simulink model "nms_3Dmodel_forward_no_rbld"  (R2017b)
settings: Solver=VariableStepAuto  StartTime=0.0  StopTime=t_end  FixedStep=1e-4  MinStep=1e-9  RelTol=1e-2  AbsTol=1e-3  EnableMultiTasking=on
InitFcn:
  | runScripts;
values from neighbouring files (symbols this model uses):
  ankle_height = 0.08    [nms_MechInit.m]
  ankleIMP = param(91+length(paramIC_opt):93+length(paramIC_opt))    [runScripts.m]
  c = 0.05    [IID_nms_MechInit.m]    (also in nms_MechInit.m)
  c_jointstop = 0.3 / (pi/180)    (= 17.1887338539)    [IID_nms_MechInit.m]    (also in nms_MechInit.m)
  CPG_On = 0    [setCPGPar.m]    (also in setCPGPar_inv.m = 1)
  CtrlPar_FP = [alpha0 alpha_cd alpha_cv]    [setCtrlPar.m]
  CtrlPar_FP_R = [R_hipR0 R_hipR_cd R_hipR_cv]    [setCtrlPar.m]
  CtrlPar_LL = l_clr    [setCtrlPar.m]
  CtrlPar_Side = [beta_cd  beta_cv]    [setCtrlPar.m]
  CtrlPar_St = [StPreStim St_M1 St_M2 St_M3 St_M4 St_M5 St_M11]    [setCtrlPar.m]
  CtrlPar_St_R = [R_StPreStim R_St_M1 R_St_M3 R_St_M4]    [setCtrlPar.m]
  CtrlPar_Sw = [SwPreStim SwPhasePari SwPhaseParii SwCtrlPar_H SwCtrlPar_A      SwCtrlPar_Ki SwCtrlPar_Kii SwCtrlPar_Kiii SwCtrlPar_StP]    [setCtrlPar.m]
  CtrlPar_Sw_R = [R_SwPreStim R_Sw_M6]    [setCtrlPar.m]
  CtrlPar_theta0 = parBlCtrl(1)      *1*pi/180    [setCtrlPar.m]
  CtrlPar_Tr = [Tr_St_sup Tr_Sw]    [setCtrlPar.m]
  CtrlPar_Tr_R = [R_Tr_St_sup R_Tr_Sw]    [setCtrlPar.m]
  D12_F = 0.16    [IID_nms_MechInit.m]    (also in nms_MechInit.m)
  D12_S = L_S    (= 0.5)    [IID_nms_MechInit.m]    (also in nms_MechInit.m = 0.46)
  D12_T = L_T    (= 0.5)    [IID_nms_MechInit.m]    (also in nms_MechInit.m = 0.46)
  D12z_T = 0.1* scalorFactor    (= 0.1)    [nms_MechInit.m]
  D13_F = 0.20    (= 0.2)    [IID_nms_MechInit.m]    (also in nms_MechInit.m)
  D1G_F = 0.14    [IID_nms_MechInit.m]    (also in nms_MechInit.m)
  D1G_HAT = 0.35    [IID_nms_MechInit.m]    (also in nms_MechInit.m)
  D1G_S = 0.3    [IID_nms_MechInit.m]    (also in nms_MechInit.m = 0.28)
  D1G_T = 0.3    [IID_nms_MechInit.m]    (also in nms_MechInit.m = 0.28)
  D1Gy_F = ankle_height*D1G_F/D12_F    (= 0.07)    [nms_MechInit.m]
  d_fBall = 0.1    [nms_MechInit.m]
  d_fHeel = 0.05    [nms_MechInit.m]
  DeltaThRef = 5e-3    (= 0.005)    [IID_nms_MechInit.m]    (also in nms_MechInit.m)
  Dist_LM23_PH = 0    [setDistPar.m]
  Dist_LM34_PH = 0    [setDistPar.m]
  Dist_On = 1    [IID_setDistPar.m]    (also in setDistPar.m)
  Dist_PDur = 0.15    [IID_setDistPar.m]    (also in setDistPar.m)
  Dist_RM23_PH = 0    [setDistPar.m]
  Dist_RM34_PH = 0    [setDistPar.m]
  Dist_StartTime = 15    [IID_setDistPar.m]    (also in setDistPar.m)
  Dist_xyzHAT_front_PH = 0    [setDistPar.m]
  Dist_xyzHAT_sag_PH = 0    [IID_setDistPar.m]    (also in setDistPar.m)
  Dist_xyzLAnkle_PH = 0    [setDistPar.m]
  Dist_xyzRAnkle_PH = 0    [setDistPar.m]
  eref = 0.04    [IID_nms_MechInit.m]    (also in nms_MechInit.m)
  FmaxBFSH = 350    [nms_MechInit.m]
  FmaxGAS = 1500    [IID_nms_MechInit.m]    (also in nms_MechInit.m)
  FmaxGLU = 1500    [IID_nms_MechInit.m]    (also in nms_MechInit.m)
  FmaxHAB = 3000    [nms_MechInit.m]
  FmaxHAD = 4500    [nms_MechInit.m]
  FmaxHAM = 3000    [IID_nms_MechInit.m]    (also in nms_MechInit.m)
  FmaxHFL = 2000    [IID_nms_MechInit.m]    (also in nms_MechInit.m)
  FmaxRF = 1200    [nms_MechInit.m]
  FmaxSOL = 4000    [IID_nms_MechInit.m]    (also in nms_MechInit.m)
  FmaxTA = 800    [IID_nms_MechInit.m]    (also in nms_MechInit.m)
  FmaxVAS = 6000    [IID_nms_MechInit.m]    (also in nms_MechInit.m)
  In_F = 0.005    [IID_nms_MechInit.m]    (also in nms_MechInit.m)
  In_HAT = 3    [IID_nms_MechInit.m]    (also in nms_MechInit.m = 2.5)
  In_S = 0.05    [IID_nms_MechInit.m]    (also in nms_MechInit.m)
  In_T = 0.15    [IID_nms_MechInit.m]    (also in nms_MechInit.m)
  init_a_tgt = 70*pi/180    (= 1.2217304764)    [setInitPar.m]
  init_a_tgtR = 90*pi/180    (= 1.57079632679)    [setInitPar.m]
  Inx_F = 0.0007    [nms_MechInit.m]
  Inx_HAT = 1.0    (= 1)    [nms_MechInit.m]
  Inx_S = 0.003    [nms_MechInit.m]
  Inx_T = 0.03    [nms_MechInit.m]
  Iny_F = 0.005    [nms_MechInit.m]
  Iny_HAT = 4.0    (= 4)    [nms_MechInit.m]
  Iny_S = 0.05    [nms_MechInit.m]
  Iny_T = 0.15    [nms_MechInit.m]
  K = 5    [IID_nms_MechInit.m]    (also in nms_MechInit.m)
  k_gn = k_gn/2    (= 39240)    [nms_MechInit.m]
  k_gt = k_gt/2    (= 3924)    [nms_MechInit.m]
  k_pressure = m_HAT * 9.81 / DeltaThRef    (= 104967)    [IID_nms_MechInit.m]    (also in nms_MechInit.m)
  leg_l = [D12_T D12_S]    [nms_MechInit.m]
  LongDelay = 0.020    (= 0.02)    [IID_setCtrlPar.m]    (also in nms_MechInit.m = 0.01)
  LongLoopDelay = 0.030    (= 0.03)    [nms_MechInit.m]
  loptBFSH = 0.12    [nms_MechInit.m]
  loptGAS = 0.05    [IID_nms_MechInit.m]    (also in nms_MechInit.m)
  loptGLU = 0.11    [IID_nms_MechInit.m]    (also in nms_MechInit.m)
  loptHAB = 0.09    [nms_MechInit.m]
  loptHAD = 0.10    (= 0.1)    [nms_MechInit.m]
  loptHAM = 0.10    (= 0.1)    [IID_nms_MechInit.m]    (also in nms_MechInit.m)
  loptHFL = 0.11    [IID_nms_MechInit.m]    (also in nms_MechInit.m)
  loptRF = 0.08    [nms_MechInit.m]
  loptSOL = 0.04    [IID_nms_MechInit.m]    (also in nms_MechInit.m)
  loptTA = 0.06    [IID_nms_MechInit.m]    (also in nms_MechInit.m)
  loptVAS = 0.08    [IID_nms_MechInit.m]    (also in nms_MechInit.m)
  lslackBFSH = 0.10    (= 0.1)    [nms_MechInit.m]
  lslackGAS = 0.40    (= 0.4)    [IID_nms_MechInit.m]    (also in nms_MechInit.m)
  lslackGLU = 0.13    [IID_nms_MechInit.m]    (also in nms_MechInit.m)
  lslackHAB = 0.07    [nms_MechInit.m]
  lslackHAD = 0.18    [nms_MechInit.m]
  lslackHAM = 0.31    [IID_nms_MechInit.m]    (also in nms_MechInit.m)
  lslackHFL = 0.10    (= 0.1)    [IID_nms_MechInit.m]    (also in nms_MechInit.m)
  lslackRF = 0.35    [nms_MechInit.m]
  lslackSOL = 0.26    [IID_nms_MechInit.m]    (also in nms_MechInit.m)
  lslackTA = 0.24    [IID_nms_MechInit.m]    (also in nms_MechInit.m)
  lslackVAS = 0.23    [IID_nms_MechInit.m]    (also in nms_MechInit.m)
  m_F = 1.25    [IID_nms_MechInit.m]    (also in nms_MechInit.m)
  m_HAT = 53.5    [IID_nms_MechInit.m]    (also in nms_MechInit.m)
  m_S = 3.5    [IID_nms_MechInit.m]    (also in nms_MechInit.m)
  m_T = 8.5    [IID_nms_MechInit.m]    (also in nms_MechInit.m)
  m_Total = m_F*2+m_S*2+m_T*2+m_HAT    (= 80)    [IID_nms_MechInit.m]    (also in nms_MechInit.m)
  massBFSH = 2    [nms_MechInit.m]
  massGAS = 0.45    [IID_nms_MechInit.m]    (also in nms_MechInit.m)
  massGLU = 1.4    [IID_nms_MechInit.m]    (also in nms_MechInit.m)
  massHAB = 1.145    [nms_MechInit.m]
  massHAD = 1.91    [nms_MechInit.m]
  massHAM = 1.82    [IID_nms_MechInit.m]    (also in nms_MechInit.m)
  massHFL = 1.87    [IID_nms_MechInit.m]    (also in nms_MechInit.m)
  massRF = 1    [nms_MechInit.m]
  massSOL = 1.36    [IID_nms_MechInit.m]    (also in nms_MechInit.m)
  massTA = 0.29    [IID_nms_MechInit.m]    (also in nms_MechInit.m)
  massVAS = 2.91    [IID_nms_MechInit.m]    (also in nms_MechInit.m)
  MidDelay = 0.010    (= 0.01)    [IID_setCtrlPar.m]    (also in nms_MechInit.m = 0.005)
  mu_slide = 0.8    [IID_nms_MechInit.m]    (also in nms_MechInit.m)
  mu_stick = 0.9    [IID_nms_MechInit.m]    (also in nms_MechInit.m)
  N = 1.5    [IID_nms_MechInit.m]    (also in cmaes_parfor.m = size(x,1); nms_MechInit.m)
  phi12_LowLimit = 70*pi/180    (= 1.2217304764)    [IID_nms_MechInit.m]    (also in nms_MechInit.m)
  phi12_UpLimit = 130*pi/180    (= 2.26892802759)    [IID_nms_MechInit.m]    (also in nms_MechInit.m)
  phi23_UpLimit = 175*pi/180    (= 3.05432619099)    [IID_nms_MechInit.m]    (also in nms_MechInit.m)
  phi34_UpLimit = 230*pi/180    (= 4.01425727959)    [IID_nms_MechInit.m]    (also in nms_MechInit.m)
  phi34R_LowLimit = -15*pi/180    (= -0.261799387799)    [nms_MechInit.m]
  ... (+115 more)
undefined symbols (not defined in the file or in its folder): magnitude, sgn
libraries: mblibv1 x104, simulink x54, simulink_extras x38, nmc x30, NMCCPG_Library x17, powerlib_meascontrol x5
(part 15 of 17)

== system nms_3Dmodel_forward_no_rbld/Neural Control Layer (Spinal Cord Control)/R Swing Phase (sagittal)/kneeii_damp and hold &kneeiii_leg stop &kneeiv_stance preparation ==
  note: Knee Phase i
  CtrlPar : Inport
  a_tgt : Inport  Port=2
  LceRF : Inport  Port=3
  LceHAM : Inport  Port=4
  VceHAM : Inport  Port=5
  VceVAS : Inport  Port=6
  VceBFSH : Inport  Port=7
  VceRF : Inport  Port=8
  LceHFL : Inport  Port=9
  LceGLU : Inport  Port=10
  LceVAS : Inport  Port=11
  Enable : EnablePort  StatesWhenEnabling=reset  ZeroCross=off
  Compare To Constant : simulink/Logic and Bit Operations/Compare To Constant  relop=<=  const=0  OutDataTypeStr=uint8  ZeroCross=off
  Constant1 : Constant  Value=0  OutDataTypeStr=boolean
  Constant2 : Constant  Value=0  OutDataTypeStr=boolean
  Constant3 : Constant  Value=0  OutDataTypeStr=boolean
  Constant4 : Constant
  Constant5 : Constant
  Demux1 : Demux  Outputs=5
  Divide1 : Product
  Divide2 : Product
  Logical Operator : Logic  Operator=NOT  AllPortsSameDT=off  OutDataTypeStr=boolean
  Logical Operator1 : Logic  AllPortsSameDT=off  OutDataTypeStr=boolean
  Relational Operator : RelationalOperator  Operator=<=  OutDataTypeStr=boolean  ZeroCross=off  RndMeth=Nearest
  Relational Operator1 : RelationalOperator  OutDataTypeStr=boolean  ZeroCross=off  RndMeth=Nearest
  S-R Flip-Flop : simulink_extras/Flip Flops/S-R Flip-Flop  initial_condition=0
  S-R Flip-Flop1 : simulink_extras/Flip Flops/S-R Flip-Flop  initial_condition=0
  S-R Flip-Flop2 : simulink_extras/Flip Flops/S-R Flip-Flop  initial_condition=0
  Sum1 : Sum  Inputs=+-|  SaturateOnIntegerOverflow=on  InputSameDT=on  OutDataTypeStr=Inherit: Same as first input
  Sum2 : Sum  Inputs=++|  SaturateOnIntegerOverflow=on  InputSameDT=on  OutDataTypeStr=Inherit: Same as first input
  Sum3 : Sum  Inputs=+-|  SaturateOnIntegerOverflow=on  InputSameDT=on  OutDataTypeStr=Inherit: Same as first input
  Sum4 : Sum  Inputs=+-|  SaturateOnIntegerOverflow=on  InputSameDT=on  OutDataTypeStr=Inherit: Same as first input
  Sum5 : Sum  Inputs=++|  SaturateOnIntegerOverflow=on  InputSameDT=on  OutDataTypeStr=Inherit: Same as first input
  Terminator : Terminator
  Terminator1 : Terminator
  Terminator2 : Terminator
  kneeii_damp and hold : Subsystem  TreatAsAtomicUnit=on
  kneeiii_leg stop : Subsystem  TreatAsAtomicUnit=on
  kneeiv_stance preparation : Subsystem  TreatAsAtomicUnit=on
  parSwKii : Selector  InputPortWidth=Sw_i  IndexOptions=Index vector (dialog)  Indices=parSwKii_i  OutputSizes=1
  parSwKiii : Selector  InputPortWidth=Sw_i  IndexOptions=Index vector (dialog)  Indices=parSwKiii_i  OutputSizes=1
  parSwKiv : Selector  InputPortWidth=Sw_i  IndexOptions=Index vector (dialog)  Indices=parSwKiv_i  OutputSizes=1
  parSwPhii : Selector  InputPortWidth=Sw_i  IndexOptions=Index vector (dialog)  Indices=parSwPhii_i  OutputSizes=1
  SRF_Sw_kii : Outport  OutputWhenDisabled=reset  InitialOutput=0
  SBFSH_Sw_kii : Outport  Port=2  OutputWhenDisabled=reset  InitialOutput=0
  SHAM_Sw_kiii : Outport  Port=3  OutputWhenDisabled=reset  InitialOutput=0
  SBFSH_Sw_kiii : Outport  Port=4  OutputWhenDisabled=reset  InitialOutput=0
  SGAS_Sw_kiii : Outport  Port=5  OutputWhenDisabled=reset  InitialOutput=0
  SHFL_Sw_kiv : Outport  Port=6  OutputWhenDisabled=reset  InitialOutput=0
  SGLU_Sw_kiv : Outport  Port=7  OutputWhenDisabled=reset  InitialOutput=0
  SVAS_Sw_kiv : Outport  Port=8  OutputWhenDisabled=reset  InitialOutput=0
  wires:
  Constant1/1 -> S-R Flip-Flop/2
  S-R Flip-Flop/2 -> Terminator/1
  Relational Operator/1 -> S-R Flip-Flop/1
  Constant2/1 -> S-R Flip-Flop1/2
  S-R Flip-Flop1/2 -> Terminator1/1
  Relational Operator1/1 -> S-R Flip-Flop1/1
  Constant3/1 -> S-R Flip-Flop2/2
  S-R Flip-Flop2/2 -> Terminator2/1
  Logical Operator1/1 -> S-R Flip-Flop2/1
  CtrlPar/1 -> parSwKii/1, parSwKiii/1, parSwKiv/1, parSwPhii/1
  S-R Flip-Flop/1 -> Logical Operator/1
  parSwKii/1 -> kneeii_damp and hold/1(CtrlPar)
  S-R Flip-Flop1/1 -> kneeiii_leg stop/Enable, Logical Operator1/1
  S-R Flip-Flop2/1 -> kneeiv_stance preparation/Enable
  parSwKiii/1 -> kneeiii_leg stop/1(CtrlPar)
  parSwKiv/1 -> kneeiv_stance preparation/1(CtrlPar)
  kneeii_damp and hold/1(SRF_Sw_kii) -> SRF_Sw_kii/1
  kneeii_damp and hold/2(SBFSH_Sw_kii) -> SBFSH_Sw_kii/1
  kneeiii_leg stop/1(SHAM_Sw_kiii) -> SHAM_Sw_kiii/1
  kneeiii_leg stop/2(SKFL_Sw_kiii) -> SBFSH_Sw_kiii/1
  kneeiii_leg stop/3(SGAS_Sw_kiii) -> SGAS_Sw_kiii/1
  kneeiv_stance preparation/1(SHFL_Sw_kiv) -> SHFL_Sw_kiv/1
  kneeiv_stance preparation/2(SGLU_Sw_kiv) -> SGLU_Sw_kiv/1
  kneeiv_stance preparation/3(SVAS_Sw_kiv) -> SVAS_Sw_kiv/1
  parSwPhii/1 -> Demux1/1
  Demux1/1 -> Sum3/2  "aRef_RF"
  Sum3/1 -> Divide1/1
  Constant4/1 -> Sum5/1
  Divide1/1 -> Sum5/2
  a_tgt/1 -> Sum2/1, Sum3/1, kneeii_damp and hold/2(a_tgt), kneeiii_leg stop/2(a_tgt), kneeiv_stance preparation/2(a_tgt)
  Demux1/2 -> Divide1/2  "a2lopt_RF"
  Sum5/1 -> Relational Operator/2  "lceOffRF"
  LceRF/1 -> kneeii_damp and hold/6(LceRF), Relational Operator/1
  Logical Operator/1 -> kneeii_damp and hold/Enable
  Demux1/3 -> Sum2/2  "a_del"
  Sum2/1 -> Sum1/1  "a_thr"
  Demux1/4 -> Sum1/2  "aRef_HAM"
  Sum1/1 -> Divide2/1
  Demux1/5 -> Divide2/2  "a2lopt_HAM"
  Constant5/1 -> Sum4/1
  Divide2/1 -> Sum4/2
  Sum4/1 -> Relational Operator1/2  "lceOffHAM"
  LceHAM/1 -> kneeiii_leg stop/3(LceHAM), Relational Operator1/1  "LceHAM"
  Compare To Constant/1 -> Logical Operator1/2
  VceHAM/1 -> Compare To Constant/1
  VceBFSH/1 -> kneeii_damp and hold/4(VceBFSH)
  VceRF/1 -> kneeii_damp and hold/5(VceRF)
  LceHFL/1 -> kneeiv_stance preparation/3(LceHFL)
  LceGLU/1 -> kneeiv_stance preparation/4(lceGLU)
  LceVAS/1 -> kneeiv_stance preparation/5(lceVAS)
  VceVAS/1 -> kneeii_damp and hold/3(VceVAS)

== system nms_3Dmodel_forward_no_rbld/Body Mechanics Layer/LLHeelCnt1/3D Contact/Friction Switch ==
  note: Static/Kinetic Friction Switch
  Slide! : Inport
  Stick! : Inport  Port=2
  Memory : Memory
  S-R Flip-Flop : simulink_extras/Flip Flops/S-R Flip-Flop  initial_condition=0
  Terminator : Terminator
  Stiction : Outport
  wires:
  Memory/1 -> Stiction/1
  Slide!/1 -> S-R Flip-Flop/2
  Stick!/1 -> S-R Flip-Flop/1
  S-R Flip-Flop/2 -> Terminator/1
  S-R Flip-Flop/1 -> Memory/1

== system nms_3Dmodel_forward_no_rbld/Body Mechanics Layer/LLHeelCnt1/3D Contact/Kinetic Friction Model ==
  note: Tangential Ground Friction
  note: Normal Ground Friction
  note: Sliding Limit Detector
  note: Footpoint Determiner
  note: Kinetic Friction Model
  vel [m/s m/s m/s] : Inport
  pos [m m m] : Inport  Port=2
  RefPt [m m m] : Inport  Port=3
  nVec [m m m] : Inport  Port=4
  Enable : EnablePort  StatesWhenEnabling=reset  ZeroCross=off
  Constant : Constant  Value=vLimit
  Constant1 : Constant  Value=[0 0 0 1]'
  Demux : Demux  Outputs=[3 1]
  FixPt Relational Operator : RelationalOperator  Operator=>  OutDataTypeStr=boolean  ZeroCross=off  RndMeth=Nearest
  Gain3 : Gain  Gain=k_gn
  Gain4 : Gain  Gain=1/v_gn_max
  Memory : Memory
  Mux1 : Mux  Inputs=2
  Mux2 : Mux  Inputs=2
  Negative : simulink/Logic and Bit Operations/Compare To Zero  relop=<  OutDataTypeStr=boolean
  Normal Axis Ground Force : Fcn  Expr="u(1)  *  (1-u(2)) * (u(2)<1)"
  Product : Product  RndMeth=Zero
  Product1 : Product  RndMeth=Zero
  Sum : Sum  Inputs=|+-
  Switch : Switch  Criteria=u2 > Threshold  Threshold=0.9*vLimit
      settings: AttributesFormatString=>%<Threshold>?
  Vector Norm : Subsystem
  d_n : DotProduct  InputSameDT=on  OutDataTypeStr=Inherit: Inherit via internal rule
  qnVec : Sum  Inputs=-+
  reverse direction : Gain  Gain=-1
  sliding friction coefficient : Gain  Gain=mu_slide
  tVec : Product  Inputs=*/  RndMeth=Zero
  v_n : DotProduct  InputSameDT=on  OutDataTypeStr=Inherit: Inherit via internal rule
  v_nVec : Product  RndMeth=Zero
  v_tVec : Sum  Inputs=-+|
  RefPtFP [m m m] : Outport  InitialOutput=[0 0 0]
      settings: AttributesFormatString=initial = '%<InitialOutput>'\nwhen disabled = '%<OutputWhenDisabled>'
  posFP [m m m] : Outport  Port=2  InitialOutput=[0 0 0]
      settings: AttributesFormatString=initial = '%<InitialOutput>'\nwhen disabled = '%<OutputWhenDisabled>'
  nVec FP [m m m] : Outport  Port=3  InitialOutput=0
      settings: AttributesFormatString=initial = '%<InitialOutput>'\nwhen disabled = '%<OutputWhenDisabled>'
  Stiction! : Outport  Port=4  OutputWhenDisabled=reset  InitialOutput=0
      settings: AttributesFormatString=initial = '%<InitialOutput>'\nwhen disabled = '%<OutputWhenDisabled>'
  F_t Slide [N N N] : Outport  Port=5  OutputWhenDisabled=reset  InitialOutput=[0 0 0]
      settings: AttributesFormatString=initial = '%<InitialOutput>'\nwhen disabled = '%<OutputWhenDisabled>'
  F_n Slide [N N N] : Outport  Port=6  OutputWhenDisabled=reset  InitialOutput=[0 0 0]
      settings: AttributesFormatString=initial = '%<InitialOutput>'\nwhen disabled = '%<OutputWhenDisabled>'
  wires:
  RefPt [m m m]/1 -> RefPtFP [m m m]/1, qnVec/2
  qnVec/1 -> d_n/1
  pos [m m m]/1 -> qnVec/1, posFP [m m m]/1
  Demux/1 -> tVec/1
  Demux/2 -> tVec/2
  Switch/1 -> Demux/1
  Mux2/1 -> Switch/1
  Constant1/1 -> Switch/3
  tVec/1 -> reverse direction/1
  Product1/1 -> F_n Slide [N N N]/1
  reverse direction/1 -> Product/2
  sliding friction coefficient/1 -> Product/1
  v_tVec/1 -> Mux2/1, Vector Norm/1(vec)
  v_nVec/1 -> v_tVec/1
  v_n/1 -> v_nVec/1, Gain4/1
  vel [m/s m/s m/s]/1 -> v_tVec/2, v_n/2
  d_n/1 -> Gain3/1
  nVec [m m m]/1 -> nVec FP [m m m]/1, Product1/1, d_n/2, v_nVec/2, v_n/1
  Gain4/1 -> Mux1/2
  Gain3/1 -> Mux1/1
  Mux1/1 -> Normal Axis Ground Force/1
  Constant/1 -> Sum/2
  Sum/1 -> Negative/1
  Vector Norm/1(norm) -> Mux2/2, Switch/2, Sum/1
  Negative/1 -> Memory/1, FixPt Relational Operator/1
  Memory/1 -> FixPt Relational Operator/2
  FixPt Relational Operator/1 -> Stiction!/1
  Product/1 -> F_t Slide [N N N]/1
  Normal Axis Ground Force/1 -> Product1/2, sliding friction coefficient/1

== system nms_3Dmodel_forward_no_rbld/Body Mechanics Layer/LLHeelCnt1/3D Contact/Static Friction Model ==
  note: Tangential Ground Reaction Force
  note: (distance to
      | surface)
  note: Zero multiplication prevents
      | horizontal friction model from
      | oscillating between static and kinetic
      | friction when the vertical force is zero but
      | the ground level is not yet reached
      | in the upward motion
  note: Static Friction Model
  note: Stiction Limit Detector
  pos [m] : Inport
  vel [m/s m/s m/s] : Inport  Port=2
  RefPtFP [m m m] : Inport  Port=3
  posFP [m] : Inport  Port=4
  nVecFP [m m m] : Inport  Port=5
  Enable : EnablePort  StatesWhenEnabling=reset  ZeroCross=off
  Abs : Abs
  Check Vertical Friction : Product  RndMeth=Zero
  Constant : Constant
  Dpos_n : DotProduct  InputSameDT=on  OutDataTypeStr=Inherit: Inherit via internal rule
  Dpos_nVec : Product  RndMeth=Zero
  Dpos_tVec : Sum  Inputs=|+-
  FixPt Relational Operator : RelationalOperator  Operator=>  OutDataTypeStr=boolean  ZeroCross=off  RndMeth=Nearest
  Gain : Gain  Gain=-1
  Gain1 : Gain  Gain=k_gn
  Gain2 : Gain  Gain=1/v_gn_max
  Gain3 : Gain  Gain=k_gt
  Gain5 : Gain  Gain=1/v_gt_max
  Memory : Memory
  Mux2 : Mux  Inputs=2
  Normal Ground Reaction Force : Fcn  Expr="u(1)  *  (1-u(2)) * (u(2)<1)"
  Positive : simulink/Logic and Bit Operations/Compare To Zero  relop=>  OutDataTypeStr=boolean
  Positive1 : simulink/Logic and Bit Operations/Compare To Zero  relop=>  OutDataTypeStr=boolean
  Product1 : Product  RndMeth=Zero
  Sign : Signum  ZeroCross=off
  Sum : Sum  Inputs=-+
  Sum1 : Sum  Inputs=|+-
  Sum2 : Sum  Inputs=|+-
  Vector Norm : Subsystem
  d_n : DotProduct  InputSameDT=on  OutDataTypeStr=Inherit: Inherit via internal rule
  stiction limit force : Gain  Gain=mu_stick
  sum : Sum  Inputs=++|
  tVec1 : Product  Inputs=**  RndMeth=Zero
  tVec2 : Product  Inputs=**  RndMeth=Zero
  v_n : DotProduct  InputSameDT=on  OutDataTypeStr=Inherit: Inherit via internal rule
  v_nVec : Product  RndMeth=Zero
  v_tVec : Sum  Inputs=-+|
  F_n Stick [N N N] : Outport  OutputWhenDisabled=reset  InitialOutput=[0 0 0]
      settings: AttributesFormatString=initial = '%<InitialOutput>'\nwhen disabled = '%<OutputWhenDisabled>'
  F_t Stick [N N N] : Outport  Port=2  OutputWhenDisabled=reset  InitialOutput=[0 0 0]
      settings: AttributesFormatString=when disabled: %<OutputWhenDisabled>\ninitial: %<InitialOutput>
  Sliding! : Outport  Port=3  OutputWhenDisabled=reset  InitialOutput=0
      settings: AttributesFormatString=when disabled: %<OutputWhenDisabled>\ninitial: %<InitialOutput>
  wires:
  Gain5/1 -> tVec1/1
  Sum1/1 -> d_n/2
  RefPtFP [m m m]/1 -> Sum1/1
  Vector Norm/1(norm) -> Sum/2
  Gain/1 -> Check Vertical Friction/1
  tVec2/1 -> Gain/1
  sum/1 -> tVec2/1
  Constant/1 -> sum/1
  tVec1/1 -> sum/2
  Sign/1 -> tVec1/2
  Gain3/1 -> tVec2/2, Sign/1
  Dpos_tVec/1 -> Gain3/1
  Dpos_nVec/1 -> Dpos_tVec/2
  Dpos_n/1 -> Dpos_nVec/2
  Sum2/1 -> Dpos_tVec/1, Dpos_n/2  "Dpos"
  posFP [m]/1 -> Sum2/2
  pos [m]/1 -> Sum1/2, Sum2/1
  Product1/1 -> F_n Stick [N N N]/1
  v_tVec/1 -> Gain5/1
  v_nVec/1 -> v_tVec/1
  v_n/1 -> Gain2/1, v_nVec/1
  vel [m/s m/s m/s]/1 -> v_n/1, v_tVec/2
  d_n/1 -> Gain1/1
  nVecFP [m m m]/1 -> Product1/1, v_nVec/2, Dpos_nVec/1, Dpos_n/1, v_n/2, d_n/1
  Gain2/1 -> Mux2/2
  Gain1/1 -> Mux2/1
  Mux2/1 -> Normal Ground Reaction Force/1
  Normal Ground Reaction Force/1 -> Positive1/1, stiction limit force/1, Product1/2
  Check Vertical Friction/1 -> F_t Stick [N N N]/1, Vector Norm/1(vec)
  Positive1/1 -> Check Vertical Friction/2
  stiction limit force/1 -> Abs/1
  Abs/1 -> Sum/1
  FixPt Relational Operator/1 -> Sliding!/1
  Positive/1 -> Memory/1, FixPt Relational Operator/1
  Memory/1 -> FixPt Relational Operator/2
  Sum/1 -> Positive/1

== system nms_3Dmodel_forward_no_rbld/Body Mechanics Layer/LLHeelCnt2/3D Contact/Friction Switch ==
  note: Static/Kinetic Friction Switch
  Slide! : Inport
  Stick! : Inport  Port=2
  Memory : Memory
  S-R Flip-Flop : simulink_extras/Flip Flops/S-R Flip-Flop  initial_condition=0
  Terminator : Terminator
  Stiction : Outport
  wires:
  Memory/1 -> Stiction/1
  Slide!/1 -> S-R Flip-Flop/2
  Stick!/1 -> S-R Flip-Flop/1
  S-R Flip-Flop/2 -> Terminator/1
  S-R Flip-Flop/1 -> Memory/1

== system nms_3Dmodel_forward_no_rbld/Body Mechanics Layer/LLHeelCnt2/3D Contact/Kinetic Friction Model ==
  note: Tangential Ground Friction
  note: Normal Ground Friction
  note: Sliding Limit Detector
  note: Footpoint Determiner
  note: Kinetic Friction Model
  vel [m/s m/s m/s] : Inport
  pos [m m m] : Inport  Port=2
  RefPt [m m m] : Inport  Port=3
  nVec [m m m] : Inport  Port=4
  Enable : EnablePort  StatesWhenEnabling=reset  ZeroCross=off
  Constant : Constant  Value=vLimit
  Constant1 : Constant  Value=[0 0 0 1]'
  Demux : Demux  Outputs=[3 1]
  FixPt Relational Operator : RelationalOperator  Operator=>  OutDataTypeStr=boolean  ZeroCross=off  RndMeth=Nearest
  Gain3 : Gain  Gain=k_gn
  Gain4 : Gain  Gain=1/v_gn_max
  Memory : Memory
  Mux1 : Mux  Inputs=2
  Mux2 : Mux  Inputs=2
  Negative : simulink/Logic and Bit Operations/Compare To Zero  relop=<  OutDataTypeStr=boolean
  Normal Axis Ground Force : Fcn  Expr="u(1)  *  (1-u(2)) * (u(2)<1)"
  Product : Product  RndMeth=Zero
  Product1 : Product  RndMeth=Zero
  Sum : Sum  Inputs=|+-
  Switch : Switch  Criteria=u2 > Threshold  Threshold=0.9*vLimit
      settings: AttributesFormatString=>%<Threshold>?
  Vector Norm : Subsystem
  d_n : DotProduct  InputSameDT=on  OutDataTypeStr=Inherit: Inherit via internal rule
  qnVec : Sum  Inputs=-+
  reverse direction : Gain  Gain=-1
  sliding friction coefficient : Gain  Gain=mu_slide
  tVec : Product  Inputs=*/  RndMeth=Zero
  v_n : DotProduct  InputSameDT=on  OutDataTypeStr=Inherit: Inherit via internal rule
  v_nVec : Product  RndMeth=Zero
  v_tVec : Sum  Inputs=-+|
  RefPtFP [m m m] : Outport  InitialOutput=[0 0 0]
      settings: AttributesFormatString=initial = '%<InitialOutput>'\nwhen disabled = '%<OutputWhenDisabled>'
  posFP [m m m] : Outport  Port=2  InitialOutput=[0 0 0]
      settings: AttributesFormatString=initial = '%<InitialOutput>'\nwhen disabled = '%<OutputWhenDisabled>'
  nVec FP [m m m] : Outport  Port=3  InitialOutput=0
      settings: AttributesFormatString=initial = '%<InitialOutput>'\nwhen disabled = '%<OutputWhenDisabled>'
  Stiction! : Outport  Port=4  OutputWhenDisabled=reset  InitialOutput=0
      settings: AttributesFormatString=initial = '%<InitialOutput>'\nwhen disabled = '%<OutputWhenDisabled>'
  F_t Slide [N N N] : Outport  Port=5  OutputWhenDisabled=reset  InitialOutput=[0 0 0]
      settings: AttributesFormatString=initial = '%<InitialOutput>'\nwhen disabled = '%<OutputWhenDisabled>'
  F_n Slide [N N N] : Outport  Port=6  OutputWhenDisabled=reset  InitialOutput=[0 0 0]
      settings: AttributesFormatString=initial = '%<InitialOutput>'\nwhen disabled = '%<OutputWhenDisabled>'
  wires:
  RefPt [m m m]/1 -> RefPtFP [m m m]/1, qnVec/2
  qnVec/1 -> d_n/1
  pos [m m m]/1 -> qnVec/1, posFP [m m m]/1
  Demux/1 -> tVec/1
  Demux/2 -> tVec/2
  Switch/1 -> Demux/1
  Mux2/1 -> Switch/1
  Constant1/1 -> Switch/3
  tVec/1 -> reverse direction/1
  Product1/1 -> F_n Slide [N N N]/1
  reverse direction/1 -> Product/2
  sliding friction coefficient/1 -> Product/1
  v_tVec/1 -> Mux2/1, Vector Norm/1(vec)
  v_nVec/1 -> v_tVec/1
  v_n/1 -> v_nVec/1, Gain4/1
  vel [m/s m/s m/s]/1 -> v_tVec/2, v_n/2
  d_n/1 -> Gain3/1
  nVec [m m m]/1 -> nVec FP [m m m]/1, Product1/1, d_n/2, v_nVec/2, v_n/1
  Gain4/1 -> Mux1/2
  Gain3/1 -> Mux1/1
  Mux1/1 -> Normal Axis Ground Force/1
  Constant/1 -> Sum/2
  Sum/1 -> Negative/1
  Vector Norm/1(norm) -> Mux2/2, Switch/2, Sum/1
  Negative/1 -> Memory/1, FixPt Relational Operator/1
  Memory/1 -> FixPt Relational Operator/2
  FixPt Relational Operator/1 -> Stiction!/1
  Product/1 -> F_t Slide [N N N]/1
  Normal Axis Ground Force/1 -> Product1/2, sliding friction coefficient/1

== system nms_3Dmodel_forward_no_rbld/Body Mechanics Layer/LLHeelCnt2/3D Contact/Static Friction Model ==
  note: Tangential Ground Reaction Force
  note: (distance to
      | surface)
  note: Zero multiplication prevents
      | horizontal friction model from
      | oscillating between static and kinetic
      | friction when the vertical force is zero but
      | the ground level is not yet reached
      | in the upward motion
  note: Static Friction Model
  note: Stiction Limit Detector
  pos [m] : Inport
  vel [m/s m/s m/s] : Inport  Port=2
  RefPtFP [m m m] : Inport  Port=3
  posFP [m] : Inport  Port=4
  nVecFP [m m m] : Inport  Port=5
  Enable : EnablePort  StatesWhenEnabling=reset  ZeroCross=off
  Abs : Abs
  Check Vertical Friction : Product  RndMeth=Zero
  Constant : Constant
  Dpos_n : DotProduct  InputSameDT=on  OutDataTypeStr=Inherit: Inherit via internal rule
  Dpos_nVec : Product  RndMeth=Zero
  Dpos_tVec : Sum  Inputs=|+-
  FixPt Relational Operator : RelationalOperator  Operator=>  OutDataTypeStr=boolean  ZeroCross=off  RndMeth=Nearest
  Gain : Gain  Gain=-1
  Gain1 : Gain  Gain=k_gn
  Gain2 : Gain  Gain=1/v_gn_max
  Gain3 : Gain  Gain=k_gt
  Gain5 : Gain  Gain=1/v_gt_max
  Memory : Memory
  Mux2 : Mux  Inputs=2
  Normal Ground Reaction Force : Fcn  Expr="u(1)  *  (1-u(2)) * (u(2)<1)"
  Positive : simulink/Logic and Bit Operations/Compare To Zero  relop=>  OutDataTypeStr=boolean
  Positive1 : simulink/Logic and Bit Operations/Compare To Zero  relop=>  OutDataTypeStr=boolean
  Product1 : Product  RndMeth=Zero
  Sign : Signum  ZeroCross=off
  Sum : Sum  Inputs=-+
  Sum1 : Sum  Inputs=|+-
  Sum2 : Sum  Inputs=|+-
  Vector Norm : Subsystem
  d_n : DotProduct  InputSameDT=on  OutDataTypeStr=Inherit: Inherit via internal rule
  stiction limit force : Gain  Gain=mu_stick
  sum : Sum  Inputs=++|
  tVec1 : Product  Inputs=**  RndMeth=Zero
  tVec2 : Product  Inputs=**  RndMeth=Zero
  v_n : DotProduct  InputSameDT=on  OutDataTypeStr=Inherit: Inherit via internal rule
  v_nVec : Product  RndMeth=Zero
  v_tVec : Sum  Inputs=-+|
  F_n Stick [N N N] : Outport  OutputWhenDisabled=reset  InitialOutput=[0 0 0]
      settings: AttributesFormatString=initial = '%<InitialOutput>'\nwhen disabled = '%<OutputWhenDisabled>'
  F_t Stick [N N N] : Outport  Port=2  OutputWhenDisabled=reset  InitialOutput=[0 0 0]
      settings: AttributesFormatString=when disabled: %<OutputWhenDisabled>\ninitial: %<InitialOutput>
  Sliding! : Outport  Port=3  OutputWhenDisabled=reset  InitialOutput=0
      settings: AttributesFormatString=when disabled: %<OutputWhenDisabled>\ninitial: %<InitialOutput>
  wires:
  Gain5/1 -> tVec1/1
  Sum1/1 -> d_n/2
  RefPtFP [m m m]/1 -> Sum1/1
  Vector Norm/1(norm) -> Sum/2
  Gain/1 -> Check Vertical Friction/1
  tVec2/1 -> Gain/1
  sum/1 -> tVec2/1
  Constant/1 -> sum/1
  tVec1/1 -> sum/2
  Sign/1 -> tVec1/2
  Gain3/1 -> tVec2/2, Sign/1
  Dpos_tVec/1 -> Gain3/1
  Dpos_nVec/1 -> Dpos_tVec/2
  Dpos_n/1 -> Dpos_nVec/2
  Sum2/1 -> Dpos_tVec/1, Dpos_n/2  "Dpos"
  posFP [m]/1 -> Sum2/2
  pos [m]/1 -> Sum1/2, Sum2/1
  Product1/1 -> F_n Stick [N N N]/1
  v_tVec/1 -> Gain5/1
  v_nVec/1 -> v_tVec/1
  v_n/1 -> Gain2/1, v_nVec/1
  vel [m/s m/s m/s]/1 -> v_n/1, v_tVec/2
  d_n/1 -> Gain1/1
  nVecFP [m m m]/1 -> Product1/1, v_nVec/2, Dpos_nVec/1, Dpos_n/1, v_n/2, d_n/1
  Gain2/1 -> Mux2/2
  Gain1/1 -> Mux2/1
  Mux2/1 -> Normal Ground Reaction Force/1
  Normal Ground Reaction Force/1 -> Positive1/1, stiction limit force/1, Product1/2
  Check Vertical Friction/1 -> F_t Stick [N N N]/1, Vector Norm/1(vec)
  Positive1/1 -> Check Vertical Friction/2
  stiction limit force/1 -> Abs/1
  Abs/1 -> Sum/1
  FixPt Relational Operator/1 -> Sliding!/1
  Positive/1 -> Memory/1, FixPt Relational Operator/1
  Memory/1 -> FixPt Relational Operator/2
  Sum/1 -> Positive/1

== system nms_3Dmodel_forward_no_rbld/Body Mechanics Layer/LLHeelCnt3/3D Contact/Friction Switch ==
  note: Static/Kinetic Friction Switch
  Slide! : Inport
  Stick! : Inport  Port=2
  Memory : Memory
  S-R Flip-Flop : simulink_extras/Flip Flops/S-R Flip-Flop  initial_condition=0
  Terminator : Terminator
  Stiction : Outport
  wires:
  S-R Flip-Flop/1 -> Memory/1
  S-R Flip-Flop/2 -> Terminator/1
  Stick!/1 -> S-R Flip-Flop/1
  Slide!/1 -> S-R Flip-Flop/2
  Memory/1 -> Stiction/1

== system nms_3Dmodel_forward_no_rbld/Body Mechanics Layer/LLHeelCnt3/3D Contact/Kinetic Friction Model ==
  note: Kinetic Friction Model
  note: Footpoint Determiner
  note: Sliding Limit Detector
  note: Normal Ground Friction
  note: Tangential Ground Friction
  vel [m/s m/s m/s] : Inport
  pos [m m m] : Inport  Port=2
  RefPt [m m m] : Inport  Port=3
  nVec [m m m] : Inport  Port=4
  Enable : EnablePort  StatesWhenEnabling=reset  ZeroCross=off
  Constant : Constant  Value=vLimit
  Constant1 : Constant  Value=[0 0 0 1]'
  Demux : Demux  Outputs=[3 1]
  FixPt Relational Operator : RelationalOperator  Operator=>  OutDataTypeStr=boolean  ZeroCross=off  RndMeth=Nearest
  Gain3 : Gain  Gain=k_gn
  Gain4 : Gain  Gain=1/v_gn_max
  Memory : Memory
  Mux1 : Mux  Inputs=2
  Mux2 : Mux  Inputs=2
  Negative : simulink/Logic and Bit Operations/Compare To Zero  relop=<  OutDataTypeStr=boolean
  Normal Axis Ground Force : Fcn  Expr="u(1)  *  (1-u(2)) * (u(2)<1)"
  Product : Product  RndMeth=Zero
  Product1 : Product  RndMeth=Zero
  Sum : Sum  Inputs=|+-
  Switch : Switch  Criteria=u2 > Threshold  Threshold=0.9*vLimit
      settings: AttributesFormatString=>%<Threshold>?
  Vector Norm : Subsystem
  d_n : DotProduct  InputSameDT=on  OutDataTypeStr=Inherit: Inherit via internal rule
  qnVec : Sum  Inputs=-+
  reverse direction : Gain  Gain=-1
  sliding friction coefficient : Gain  Gain=mu_slide
  tVec : Product  Inputs=*/  RndMeth=Zero
  v_n : DotProduct  InputSameDT=on  OutDataTypeStr=Inherit: Inherit via internal rule
  v_nVec : Product  RndMeth=Zero
  v_tVec : Sum  Inputs=-+|
  RefPtFP [m m m] : Outport  InitialOutput=[0 0 0]
      settings: AttributesFormatString=initial = '%<InitialOutput>'\nwhen disabled = '%<OutputWhenDisabled>'
  posFP [m m m] : Outport  Port=2  InitialOutput=[0 0 0]
      settings: AttributesFormatString=initial = '%<InitialOutput>'\nwhen disabled = '%<OutputWhenDisabled>'
  nVec FP [m m m] : Outport  Port=3  InitialOutput=0
      settings: AttributesFormatString=initial = '%<InitialOutput>'\nwhen disabled = '%<OutputWhenDisabled>'
  Stiction! : Outport  Port=4  OutputWhenDisabled=reset  InitialOutput=0
      settings: AttributesFormatString=initial = '%<InitialOutput>'\nwhen disabled = '%<OutputWhenDisabled>'
  F_t Slide [N N N] : Outport  Port=5  OutputWhenDisabled=reset  InitialOutput=[0 0 0]
      settings: AttributesFormatString=initial = '%<InitialOutput>'\nwhen disabled = '%<OutputWhenDisabled>'
  F_n Slide [N N N] : Outport  Port=6  OutputWhenDisabled=reset  InitialOutput=[0 0 0]
      settings: AttributesFormatString=initial = '%<InitialOutput>'\nwhen disabled = '%<OutputWhenDisabled>'
  wires:
  Normal Axis Ground Force/1 -> sliding friction coefficient/1, Product1/2
  Product/1 -> F_t Slide [N N N]/1
  FixPt Relational Operator/1 -> Stiction!/1
  Memory/1 -> FixPt Relational Operator/2
  Negative/1 -> FixPt Relational Operator/1, Memory/1
  Vector Norm/1(norm) -> Sum/1, Switch/2, Mux2/2
  Sum/1 -> Negative/1
  Constant/1 -> Sum/2
  Mux1/1 -> Normal Axis Ground Force/1
  Gain3/1 -> Mux1/1
  Gain4/1 -> Mux1/2
  nVec [m m m]/1 -> v_n/1, v_nVec/2, d_n/2, Product1/1, nVec FP [m m m]/1
  d_n/1 -> Gain3/1
  vel [m/s m/s m/s]/1 -> v_n/2, v_tVec/2
  v_n/1 -> Gain4/1, v_nVec/1
  v_nVec/1 -> v_tVec/1
  v_tVec/1 -> Vector Norm/1(vec), Mux2/1
  sliding friction coefficient/1 -> Product/1
  reverse direction/1 -> Product/2
  Product1/1 -> F_n Slide [N N N]/1
  tVec/1 -> reverse direction/1
  Constant1/1 -> Switch/3
  Mux2/1 -> Switch/1
  Switch/1 -> Demux/1
  Demux/2 -> tVec/2
  Demux/1 -> tVec/1
  pos [m m m]/1 -> posFP [m m m]/1, qnVec/1
  qnVec/1 -> d_n/1
  RefPt [m m m]/1 -> qnVec/2, RefPtFP [m m m]/1

== system nms_3Dmodel_forward_no_rbld/Body Mechanics Layer/LLHeelCnt3/3D Contact/Static Friction Model ==
  note: Stiction Limit Detector
  note: Static Friction Model
  note: Zero multiplication prevents
      | horizontal friction model from
      | oscillating between static and kinetic
      | friction when the vertical force is zero but
      | the ground level is not yet reached
      | in the upward motion
  note: (distance to
      | surface)
  note: Tangential Ground Reaction Force
  pos [m] : Inport
  vel [m/s m/s m/s] : Inport  Port=2
  RefPtFP [m m m] : Inport  Port=3
  posFP [m] : Inport  Port=4
  nVecFP [m m m] : Inport  Port=5
  Enable : EnablePort  StatesWhenEnabling=reset  ZeroCross=off
  Abs : Abs
  Check Vertical Friction : Product  RndMeth=Zero
  Constant : Constant
  Dpos_n : DotProduct  InputSameDT=on  OutDataTypeStr=Inherit: Inherit via internal rule
  Dpos_nVec : Product  RndMeth=Zero
  Dpos_tVec : Sum  Inputs=|+-
  FixPt Relational Operator : RelationalOperator  Operator=>  OutDataTypeStr=boolean  ZeroCross=off  RndMeth=Nearest
  Gain : Gain  Gain=-1
  Gain1 : Gain  Gain=k_gn
  Gain2 : Gain  Gain=1/v_gn_max
  Gain3 : Gain  Gain=k_gt
  Gain5 : Gain  Gain=1/v_gt_max
  Memory : Memory
  Mux2 : Mux  Inputs=2
  Normal Ground Reaction Force : Fcn  Expr="u(1)  *  (1-u(2)) * (u(2)<1)"
  Positive : simulink/Logic and Bit Operations/Compare To Zero  relop=>  OutDataTypeStr=boolean
  Positive1 : simulink/Logic and Bit Operations/Compare To Zero  relop=>  OutDataTypeStr=boolean
  Product1 : Product  RndMeth=Zero
  Sign : Signum  ZeroCross=off
  Sum : Sum  Inputs=-+
  Sum1 : Sum  Inputs=|+-
  Sum2 : Sum  Inputs=|+-
  Vector Norm : Subsystem
  d_n : DotProduct  InputSameDT=on  OutDataTypeStr=Inherit: Inherit via internal rule
  stiction limit force : Gain  Gain=mu_stick
  sum : Sum  Inputs=++|
  tVec1 : Product  Inputs=**  RndMeth=Zero
  tVec2 : Product  Inputs=**  RndMeth=Zero
  v_n : DotProduct  InputSameDT=on  OutDataTypeStr=Inherit: Inherit via internal rule
  v_nVec : Product  RndMeth=Zero
  v_tVec : Sum  Inputs=-+|
  F_n Stick [N N N] : Outport  OutputWhenDisabled=reset  InitialOutput=[0 0 0]
      settings: AttributesFormatString=initial = '%<InitialOutput>'\nwhen disabled = '%<OutputWhenDisabled>'
  F_t Stick [N N N] : Outport  Port=2  OutputWhenDisabled=reset  InitialOutput=[0 0 0]
      settings: AttributesFormatString=when disabled: %<OutputWhenDisabled>\ninitial: %<InitialOutput>
  Sliding! : Outport  Port=3  OutputWhenDisabled=reset  InitialOutput=0
      settings: AttributesFormatString=when disabled: %<OutputWhenDisabled>\ninitial: %<InitialOutput>
  wires:
  Sum/1 -> Positive/1
  Memory/1 -> FixPt Relational Operator/2
  Positive/1 -> FixPt Relational Operator/1, Memory/1
  FixPt Relational Operator/1 -> Sliding!/1
  Abs/1 -> Sum/1
  stiction limit force/1 -> Abs/1
  Positive1/1 -> Check Vertical Friction/2
  Check Vertical Friction/1 -> Vector Norm/1(vec), F_t Stick [N N N]/1
  Normal Ground Reaction Force/1 -> Product1/2, stiction limit force/1, Positive1/1
  Mux2/1 -> Normal Ground Reaction Force/1
  Gain1/1 -> Mux2/1
  Gain2/1 -> Mux2/2
  nVecFP [m m m]/1 -> d_n/1, v_n/2, Dpos_n/1, Dpos_nVec/1, v_nVec/2, Product1/1
  d_n/1 -> Gain1/1
  vel [m/s m/s m/s]/1 -> v_tVec/2, v_n/1
  v_n/1 -> v_nVec/1, Gain2/1
  v_nVec/1 -> v_tVec/1
  v_tVec/1 -> Gain5/1
  Product1/1 -> F_n Stick [N N N]/1
  pos [m]/1 -> Sum2/1, Sum1/2
  posFP [m]/1 -> Sum2/2
  Sum2/1 -> Dpos_n/2, Dpos_tVec/1  "Dpos"
  Dpos_n/1 -> Dpos_nVec/2
  Dpos_nVec/1 -> Dpos_tVec/2
  Dpos_tVec/1 -> Gain3/1
  Gain3/1 -> Sign/1, tVec2/2
  Sign/1 -> tVec1/2
  tVec1/1 -> sum/2
  Constant/1 -> sum/1
  sum/1 -> tVec2/1
  tVec2/1 -> Gain/1
  Gain/1 -> Check Vertical Friction/1
  Vector Norm/1(norm) -> Sum/2
  RefPtFP [m m m]/1 -> Sum1/1
  Sum1/1 -> d_n/2
  Gain5/1 -> tVec1/1

== system nms_3Dmodel_forward_no_rbld/Body Mechanics Layer/LLHeelCnt4/3D Contact/Friction Switch ==
  note: Static/Kinetic Friction Switch
  Slide! : Inport
  Stick! : Inport  Port=2
  Memory : Memory
  S-R Flip-Flop : simulink_extras/Flip Flops/S-R Flip-Flop  initial_condition=0
  Terminator : Terminator
  Stiction : Outport
  wires:
  S-R Flip-Flop/1 -> Memory/1
  S-R Flip-Flop/2 -> Terminator/1
  Stick!/1 -> S-R Flip-Flop/1
  Slide!/1 -> S-R Flip-Flop/2
  Memory/1 -> Stiction/1

== system nms_3Dmodel_forward_no_rbld/Body Mechanics Layer/LLHeelCnt4/3D Contact/Kinetic Friction Model ==
  note: Kinetic Friction Model
  note: Footpoint Determiner
  note: Sliding Limit Detector
  note: Normal Ground Friction
  note: Tangential Ground Friction
  vel [m/s m/s m/s] : Inport
  pos [m m m] : Inport  Port=2
  RefPt [m m m] : Inport  Port=3
  nVec [m m m] : Inport  Port=4
  Enable : EnablePort  StatesWhenEnabling=reset  ZeroCross=off
  Constant : Constant  Value=vLimit
  Constant1 : Constant  Value=[0 0 0 1]'
  Demux : Demux  Outputs=[3 1]
  FixPt Relational Operator : RelationalOperator  Operator=>  OutDataTypeStr=boolean  ZeroCross=off  RndMeth=Nearest
  Gain3 : Gain  Gain=k_gn
  Gain4 : Gain  Gain=1/v_gn_max
  Memory : Memory
  Mux1 : Mux  Inputs=2
  Mux2 : Mux  Inputs=2
  Negative : simulink/Logic and Bit Operations/Compare To Zero  relop=<  OutDataTypeStr=boolean
  Normal Axis Ground Force : Fcn  Expr="u(1)  *  (1-u(2)) * (u(2)<1)"
  Product : Product  RndMeth=Zero
  Product1 : Product  RndMeth=Zero
  Sum : Sum  Inputs=|+-
  Switch : Switch  Criteria=u2 > Threshold  Threshold=0.9*vLimit
      settings: AttributesFormatString=>%<Threshold>?
  Vector Norm : Subsystem
  d_n : DotProduct  InputSameDT=on  OutDataTypeStr=Inherit: Inherit via internal rule
  qnVec : Sum  Inputs=-+
  reverse direction : Gain  Gain=-1
  sliding friction coefficient : Gain  Gain=mu_slide
  tVec : Product  Inputs=*/  RndMeth=Zero
  v_n : DotProduct  InputSameDT=on  OutDataTypeStr=Inherit: Inherit via internal rule
  v_nVec : Product  RndMeth=Zero
  v_tVec : Sum  Inputs=-+|
  RefPtFP [m m m] : Outport  InitialOutput=[0 0 0]
      settings: AttributesFormatString=initial = '%<InitialOutput>'\nwhen disabled = '%<OutputWhenDisabled>'
  posFP [m m m] : Outport  Port=2  InitialOutput=[0 0 0]
      settings: AttributesFormatString=initial = '%<InitialOutput>'\nwhen disabled = '%<OutputWhenDisabled>'
  nVec FP [m m m] : Outport  Port=3  InitialOutput=0
      settings: AttributesFormatString=initial = '%<InitialOutput>'\nwhen disabled = '%<OutputWhenDisabled>'
  Stiction! : Outport  Port=4  OutputWhenDisabled=reset  InitialOutput=0
      settings: AttributesFormatString=initial = '%<InitialOutput>'\nwhen disabled = '%<OutputWhenDisabled>'
  F_t Slide [N N N] : Outport  Port=5  OutputWhenDisabled=reset  InitialOutput=[0 0 0]
      settings: AttributesFormatString=initial = '%<InitialOutput>'\nwhen disabled = '%<OutputWhenDisabled>'
  F_n Slide [N N N] : Outport  Port=6  OutputWhenDisabled=reset  InitialOutput=[0 0 0]
      settings: AttributesFormatString=initial = '%<InitialOutput>'\nwhen disabled = '%<OutputWhenDisabled>'
  wires:
  Normal Axis Ground Force/1 -> sliding friction coefficient/1, Product1/2
  Product/1 -> F_t Slide [N N N]/1
  FixPt Relational Operator/1 -> Stiction!/1
  Memory/1 -> FixPt Relational Operator/2
  Negative/1 -> FixPt Relational Operator/1, Memory/1
  Vector Norm/1(norm) -> Sum/1, Switch/2, Mux2/2
  Sum/1 -> Negative/1
  Constant/1 -> Sum/2
  Mux1/1 -> Normal Axis Ground Force/1
  Gain3/1 -> Mux1/1
  Gain4/1 -> Mux1/2
  nVec [m m m]/1 -> v_n/1, v_nVec/2, d_n/2, Product1/1, nVec FP [m m m]/1
  d_n/1 -> Gain3/1
  vel [m/s m/s m/s]/1 -> v_n/2, v_tVec/2
  v_n/1 -> Gain4/1, v_nVec/1
  v_nVec/1 -> v_tVec/1
  v_tVec/1 -> Vector Norm/1(vec), Mux2/1
  sliding friction coefficient/1 -> Product/1
  reverse direction/1 -> Product/2
  Product1/1 -> F_n Slide [N N N]/1
  tVec/1 -> reverse direction/1
  Constant1/1 -> Switch/3
  Mux2/1 -> Switch/1
  Switch/1 -> Demux/1
  Demux/2 -> tVec/2
  Demux/1 -> tVec/1
  pos [m m m]/1 -> posFP [m m m]/1, qnVec/1
  qnVec/1 -> d_n/1
  RefPt [m m m]/1 -> qnVec/2, RefPtFP [m m m]/1

== system nms_3Dmodel_forward_no_rbld/Body Mechanics Layer/LLHeelCnt4/3D Contact/Static Friction Model ==
  note: Stiction Limit Detector
  note: Static Friction Model
  note: Zero multiplication prevents
      | horizontal friction model from
      | oscillating between static and kinetic
      | friction when the vertical force is zero but
      | the ground level is not yet reached
      | in the upward motion
  note: (distance to
      | surface)
  note: Tangential Ground Reaction Force
  pos [m] : Inport
  vel [m/s m/s m/s] : Inport  Port=2
  RefPtFP [m m m] : Inport  Port=3
  posFP [m] : Inport  Port=4
  nVecFP [m m m] : Inport  Port=5
  Enable : EnablePort  StatesWhenEnabling=reset  ZeroCross=off
  Abs : Abs
  Check Vertical Friction : Product  RndMeth=Zero
  Constant : Constant
  Dpos_n : DotProduct  InputSameDT=on  OutDataTypeStr=Inherit: Inherit via internal rule
  Dpos_nVec : Product  RndMeth=Zero
  Dpos_tVec : Sum  Inputs=|+-
  FixPt Relational Operator : RelationalOperator  Operator=>  OutDataTypeStr=boolean  ZeroCross=off  RndMeth=Nearest
  Gain : Gain  Gain=-1
  Gain1 : Gain  Gain=k_gn
  Gain2 : Gain  Gain=1/v_gn_max
  Gain3 : Gain  Gain=k_gt
  Gain5 : Gain  Gain=1/v_gt_max
  Memory : Memory
  Mux2 : Mux  Inputs=2
  Normal Ground Reaction Force : Fcn  Expr="u(1)  *  (1-u(2)) * (u(2)<1)"
  Positive : simulink/Logic and Bit Operations/Compare To Zero  relop=>  OutDataTypeStr=boolean
  Positive1 : simulink/Logic and Bit Operations/Compare To Zero  relop=>  OutDataTypeStr=boolean
  Product1 : Product  RndMeth=Zero
  Sign : Signum  ZeroCross=off
  Sum : Sum  Inputs=-+
  Sum1 : Sum  Inputs=|+-
  Sum2 : Sum  Inputs=|+-
  Vector Norm : Subsystem
  d_n : DotProduct  InputSameDT=on  OutDataTypeStr=Inherit: Inherit via internal rule
  stiction limit force : Gain  Gain=mu_stick
  sum : Sum  Inputs=++|
  tVec1 : Product  Inputs=**  RndMeth=Zero
  tVec2 : Product  Inputs=**  RndMeth=Zero
  v_n : DotProduct  InputSameDT=on  OutDataTypeStr=Inherit: Inherit via internal rule
  v_nVec : Product  RndMeth=Zero
  v_tVec : Sum  Inputs=-+|
  F_n Stick [N N N] : Outport  OutputWhenDisabled=reset  InitialOutput=[0 0 0]
      settings: AttributesFormatString=initial = '%<InitialOutput>'\nwhen disabled = '%<OutputWhenDisabled>'
  F_t Stick [N N N] : Outport  Port=2  OutputWhenDisabled=reset  InitialOutput=[0 0 0]
      settings: AttributesFormatString=when disabled: %<OutputWhenDisabled>\ninitial: %<InitialOutput>
  Sliding! : Outport  Port=3  OutputWhenDisabled=reset  InitialOutput=0
      settings: AttributesFormatString=when disabled: %<OutputWhenDisabled>\ninitial: %<InitialOutput>
  wires:
  Sum/1 -> Positive/1
  Memory/1 -> FixPt Relational Operator/2
  Positive/1 -> FixPt Relational Operator/1, Memory/1
  FixPt Relational Operator/1 -> Sliding!/1
  Abs/1 -> Sum/1
  stiction limit force/1 -> Abs/1
  Positive1/1 -> Check Vertical Friction/2
  Check Vertical Friction/1 -> Vector Norm/1(vec), F_t Stick [N N N]/1
  Normal Ground Reaction Force/1 -> Product1/2, stiction limit force/1, Positive1/1
  Mux2/1 -> Normal Ground Reaction Force/1
  Gain1/1 -> Mux2/1
  Gain2/1 -> Mux2/2
  nVecFP [m m m]/1 -> d_n/1, v_n/2, Dpos_n/1, Dpos_nVec/1, v_nVec/2, Product1/1
  d_n/1 -> Gain1/1
  vel [m/s m/s m/s]/1 -> v_tVec/2, v_n/1
  v_n/1 -> v_nVec/1, Gain2/1
  v_nVec/1 -> v_tVec/1
  v_tVec/1 -> Gain5/1
  Product1/1 -> F_n Stick [N N N]/1
  pos [m]/1 -> Sum2/1, Sum1/2
  posFP [m]/1 -> Sum2/2
  Sum2/1 -> Dpos_n/2, Dpos_tVec/1  "Dpos"
  Dpos_n/1 -> Dpos_nVec/2
  Dpos_nVec/1 -> Dpos_tVec/2
  Dpos_tVec/1 -> Gain3/1
  Gain3/1 -> Sign/1, tVec2/2
  Sign/1 -> tVec1/2
  tVec1/1 -> sum/2
  Constant/1 -> sum/1
  sum/1 -> tVec2/1
  tVec2/1 -> Gain/1
  Gain/1 -> Check Vertical Friction/1
  Vector Norm/1(norm) -> Sum/2
  RefPtFP [m m m]/1 -> Sum1/1
  Sum1/1 -> d_n/2
  Gain5/1 -> tVec1/1

== system nms_3Dmodel_forward_no_rbld/Body Mechanics Layer/LLHeelCnt5/3D Contact/Friction Switch ==
  note: Static/Kinetic Friction Switch
  Slide! : Inport
  Stick! : Inport  Port=2
  Memory : Memory
  S-R Flip-Flop : simulink_extras/Flip Flops/S-R Flip-Flop  initial_condition=0
  Terminator : Terminator
  Stiction : Outport
  wires:
  Memory/1 -> Stiction/1
  Slide!/1 -> S-R Flip-Flop/2
  Stick!/1 -> S-R Flip-Flop/1
  S-R Flip-Flop/2 -> Terminator/1
  S-R Flip-Flop/1 -> Memory/1

== system nms_3Dmodel_forward_no_rbld/Body Mechanics Layer/LLHeelCnt5/3D Contact/Kinetic Friction Model ==
  note: Tangential Ground Friction
  note: Normal Ground Friction
  note: Sliding Limit Detector
  note: Footpoint Determiner
  note: Kinetic Friction Model
  vel [m/s m/s m/s] : Inport
  pos [m m m] : Inport  Port=2
  RefPt [m m m] : Inport  Port=3
  nVec [m m m] : Inport  Port=4
  Enable : EnablePort  StatesWhenEnabling=reset  ZeroCross=off
  Constant : Constant  Value=vLimit
  Constant1 : Constant  Value=[0 0 0 1]'
  Demux : Demux  Outputs=[3 1]
  FixPt Relational Operator : RelationalOperator  Operator=>  OutDataTypeStr=boolean  ZeroCross=off  RndMeth=Nearest
  Gain3 : Gain  Gain=k_gn
  Gain4 : Gain  Gain=1/v_gn_max
  Memory : Memory
  Mux1 : Mux  Inputs=2
  Mux2 : Mux  Inputs=2
  Negative : simulink/Logic and Bit Operations/Compare To Zero  relop=<  OutDataTypeStr=boolean
  Normal Axis Ground Force : Fcn  Expr="u(1)  *  (1-u(2)) * (u(2)<1)"
  Product : Product  RndMeth=Zero
  Product1 : Product  RndMeth=Zero
  Sum : Sum  Inputs=|+-
  Switch : Switch  Criteria=u2 > Threshold  Threshold=0.9*vLimit
      settings: AttributesFormatString=>%<Threshold>?
  Vector Norm : Subsystem
  d_n : DotProduct  InputSameDT=on  OutDataTypeStr=Inherit: Inherit via internal rule
  qnVec : Sum  Inputs=-+
  reverse direction : Gain  Gain=-1
  sliding friction coefficient : Gain  Gain=mu_slide
  tVec : Product  Inputs=*/  RndMeth=Zero
  v_n : DotProduct  InputSameDT=on  OutDataTypeStr=Inherit: Inherit via internal rule
  v_nVec : Product  RndMeth=Zero
  v_tVec : Sum  Inputs=-+|
  RefPtFP [m m m] : Outport  InitialOutput=[0 0 0]
      settings: AttributesFormatString=initial = '%<InitialOutput>'\nwhen disabled = '%<OutputWhenDisabled>'
  posFP [m m m] : Outport  Port=2  InitialOutput=[0 0 0]
      settings: AttributesFormatString=initial = '%<InitialOutput>'\nwhen disabled = '%<OutputWhenDisabled>'
  nVec FP [m m m] : Outport  Port=3  InitialOutput=0
      settings: AttributesFormatString=initial = '%<InitialOutput>'\nwhen disabled = '%<OutputWhenDisabled>'
  Stiction! : Outport  Port=4  OutputWhenDisabled=reset  InitialOutput=0
      settings: AttributesFormatString=initial = '%<InitialOutput>'\nwhen disabled = '%<OutputWhenDisabled>'
  F_t Slide [N N N] : Outport  Port=5  OutputWhenDisabled=reset  InitialOutput=[0 0 0]
      settings: AttributesFormatString=initial = '%<InitialOutput>'\nwhen disabled = '%<OutputWhenDisabled>'
  F_n Slide [N N N] : Outport  Port=6  OutputWhenDisabled=reset  InitialOutput=[0 0 0]
      settings: AttributesFormatString=initial = '%<InitialOutput>'\nwhen disabled = '%<OutputWhenDisabled>'
  wires:
  RefPt [m m m]/1 -> RefPtFP [m m m]/1, qnVec/2
  qnVec/1 -> d_n/1
  pos [m m m]/1 -> qnVec/1, posFP [m m m]/1
  Demux/1 -> tVec/1
  Demux/2 -> tVec/2
  Switch/1 -> Demux/1
  Mux2/1 -> Switch/1
  Constant1/1 -> Switch/3
  tVec/1 -> reverse direction/1
  Product1/1 -> F_n Slide [N N N]/1
  reverse direction/1 -> Product/2
  sliding friction coefficient/1 -> Product/1
  v_tVec/1 -> Mux2/1, Vector Norm/1(vec)
  v_nVec/1 -> v_tVec/1
  v_n/1 -> v_nVec/1, Gain4/1
  vel [m/s m/s m/s]/1 -> v_tVec/2, v_n/2
  d_n/1 -> Gain3/1
  nVec [m m m]/1 -> nVec FP [m m m]/1, Product1/1, d_n/2, v_nVec/2, v_n/1
  Gain4/1 -> Mux1/2
  Gain3/1 -> Mux1/1
  Mux1/1 -> Normal Axis Ground Force/1
  Constant/1 -> Sum/2
  Sum/1 -> Negative/1
  Vector Norm/1(norm) -> Mux2/2, Switch/2, Sum/1
  Negative/1 -> Memory/1, FixPt Relational Operator/1
  Memory/1 -> FixPt Relational Operator/2
  FixPt Relational Operator/1 -> Stiction!/1
  Product/1 -> F_t Slide [N N N]/1
  Normal Axis Ground Force/1 -> Product1/2, sliding friction coefficient/1
